simulink library "INT_Fans_ClgDem"  (R2016b)
settings: Solver=VariableStepAuto  StartTime=0.0  StopTime=10.0  RelTol=1e-3
settings Model: Creator=xinchangran  LastModifiedBy=xinchangran

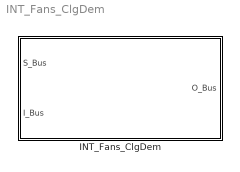
== system INT_Fans_ClgDem ==
  INT_Fans_ClgDem : Subsystem

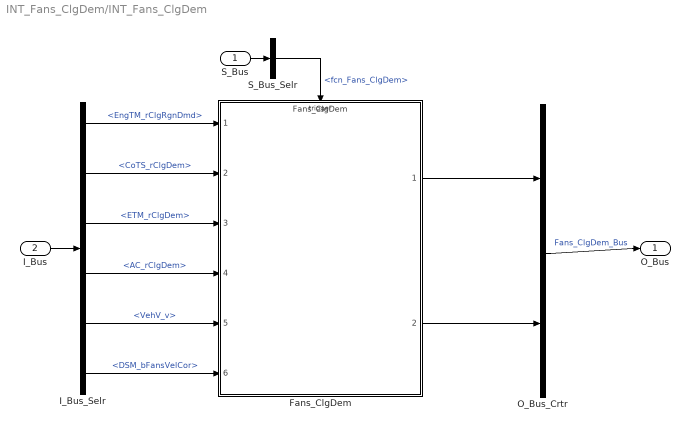
== system INT_Fans_ClgDem/INT_Fans_ClgDem ==
  S_Bus : Inport
  I_Bus : Inport  Port=2
  Fans_ClgDem : ModelReference  ModelNameDialog=Fans_ClgDem  SimulationMode=Normal  ModelReferenceVersion=1.41  TriggerPortName=function  TriggerPortTriggerType=function-call  TriggerPortStatesWhenEnabling=held
  I_Bus_Selr : BusSelector  OutputSignals=EngTM_rClgRgnDmd,CoTS_rClgDem,ETM_rClgDem,AC_rClgDem,VehV_v,DSM_bFansVelCor
  O_Bus_Crtr : BusCreator  Inputs=2
  S_Bus_Selr : BusSelector  OutputSignals=fcn_Fans_ClgDem
  O_Bus : Outport
  wires:
  S_Bus_Selr/1 -> Fans_ClgDem/Trigger  "<fcn_Fans_ClgDem>"
  S_Bus/1 -> S_Bus_Selr/1
  I_Bus/1 -> I_Bus_Selr/1
  I_Bus_Selr/1 -> Fans_ClgDem/1  "<EngTM_rClgRgnDmd>"
  I_Bus_Selr/2 -> Fans_ClgDem/2  "<CoTS_rClgDem>"
  I_Bus_Selr/3 -> Fans_ClgDem/3  "<ETM_rClgDem>"
  I_Bus_Selr/4 -> Fans_ClgDem/4  "<AC_rClgDem>"
  I_Bus_Selr/5 -> Fans_ClgDem/5  "<VehV_v>"
  I_Bus_Selr/6 -> Fans_ClgDem/6  "<DSM_bFansVelCor>"
  O_Bus_Crtr/1 -> O_Bus/1  "Fans_ClgDem_Bus"
  Fans_ClgDem/1 -> O_Bus_Crtr/1
  Fans_ClgDem/2 -> O_Bus_Crtr/2
